simulink library "asbhl20FADEC"  (R2016b)
settings: Solver=VariableStepAuto  StartTime=0.0  StopTime=10.0  RelTol=1e-3
undefined symbols (not defined in the file): Tc
Description:
  | HL-20 propulsion system control component module (stub)
  | 
  | Copyright 1990-2005 The MathWorks Inc.
settings Model: Creator=The MathWorks, Inc.  LastModifiedBy=The MathWorks, Inc.
settings DataIOCC: SaveFormat=Array  SignalLoggingSaveFormat=ModelDataLogs
settings OptimizationCC: BlockReduction=off  BooleanDataType=off
settings DebuggingCC: SaveWithParameterizedLinksMsg=none  UnderspecifiedInitializationDetection=Classic  MergeDetectMultiDrivingBlocksExec=none  SignalResolutionControl=TryResolveAllWithWarning  MultiTaskCondExecSysMsg=none  StrictBusMsg=None
settings HardwareCC: ProdBitPerPointer=32  ProdBitPerSizeT=32  ProdBitPerPtrDiffT=32  ProdLargestAtomicFloat=None  ProdIntDivRoundTo=Undefined  ProdEndianess=Unspecified  ProdWordSize=32  ProdHWDeviceType=32-bit Generic  TargetUnknown=on
settings ModelReferenceCC: PropagateSignalLabelsOutOfModel=off
settings ConfigComp: CovMetricSettings=dw  CovHtmlReporting=on  CovSaveCumulativeToWorkspaceVar=on  CovSaveSingleToWorkspaceVar=on  CovExternalEMLEnable=off

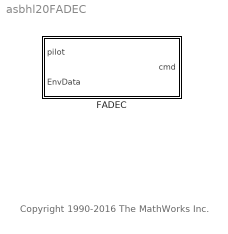
== system asbhl20FADEC ==
  note: Copyright 1990-2016 The MathWorks Inc.
  FADEC : Subsystem  TreatAsAtomicUnit=on

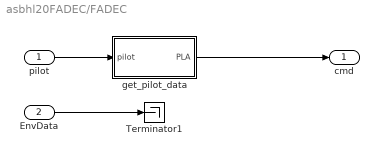
== system asbhl20FADEC/FADEC ==
  pilot : Inport
  EnvData : Inport  Port=2
  Terminator1 : Terminator
  get_pilot_data : Subsystem
  cmd : Outport
  wires:
  pilot/1 -> get_pilot_data/1(pilot)
  get_pilot_data/1(PLA) -> cmd/1
  EnvData/1 -> Terminator1/1

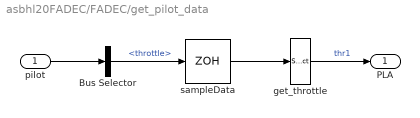
== system asbhl20FADEC/FADEC/get_pilot_data ==
  pilot : Inport
  Bus Selector : BusSelector  OutputSignals=throttle
  get_throttle : Selector  InputPortWidth=4  IndexOptions=Index vector (dialog)  Indices=1  OutputSizes=1
  sampleData : ZeroOrderHold  SampleTime=Tc
  PLA : Outport
  wires:
  Bus Selector/1 -> sampleData/1  "<throttle>"
  pilot/1 -> Bus Selector/1
  get_throttle/1 -> PLA/1  "thr1"
  sampleData/1 -> get_throttle/1
